simulink model "ADRC_DaoLiBai_test"  (R2018b)
settings: Solver=VariableStepAuto  StartTime=0.0  StopTime=10.0  RelTol=1e-3
settings Model: Creator=ILQMN  LastModifiedBy=ILQMN

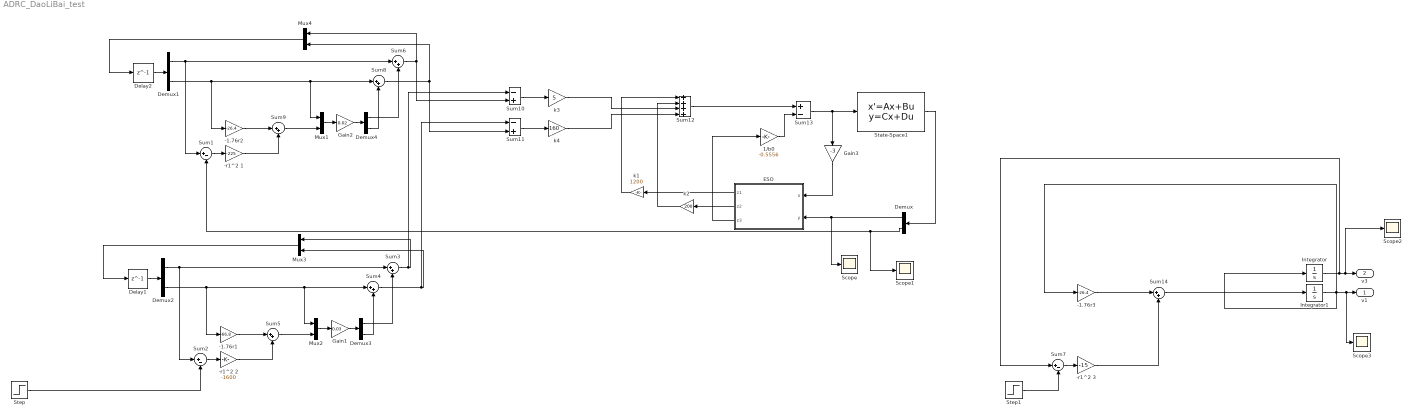
== system ADRC_DaoLiBai_test ==
  -1.76r1 : Gain  Gain=-66.8
  -1.76r2 : Gain  Gain=-26.4
  -1.76r3 : Gain  Gain=-26.4
  -r1^2 1 : Gain  Gain=-225
  -r1^2 2 : Gain  Gain=-1600
  -r1^2 3 : Gain  Gain=-15
  "1/b0 " : Gain  Gain=-0.5556
  Delay1 : Delay  DelayLength=1
  Delay2 : Delay  DelayLength=1
  Demux{,1..4} (5 alike) : Demux  Outputs=2
  ESO : Subsystem
  Gain1 : Gain  Gain=0.03
  Gain2 : Gain  Gain=0.02
  Gain3 : Gain  Gain=-3
  Integrator : Integrator
  Integrator1 : Integrator
  Mux{1..4} (4 alike) : Mux  Inputs=2
  Scope{,1..3} (4 alike) : Scope
  State-Space1 : StateSpace  A=[0 1 0 0;27.828 0 0 -0.2357;0 0 0 1;0.6393 0 0 -0.08832]  B=[0;2.6683;0;0.8832]  C=[1 0 0 0;0 0 1 0]  D=[0;0]  InitialCondition=[0;0;0;0]
  Step : Step  Time=2  After=0.2  SampleTime=0
  Step1 : Step  Time=0  SampleTime=0
  Sum1 : Sum  Inputs=|+-
  Sum10 : Sum  Inputs=-+
  Sum11 : Sum  Inputs=-+
  Sum12 : Sum  Inputs=++++
  Sum13 : Sum  Inputs=+-
  Sum{3..6,8..9,14} (7 alike) : Sum  Inputs=|++
  Sum2 : Sum  Inputs=|+-
  Sum7 : Sum  Inputs=|+-
  k1 : Gain  Gain=1200
  k2 : Gain  Gain=200
  k3 : Gain  Gain=5
  "k4 " : Gain  Gain=160
  v1 : Outport
  v3 : Outport  Port=2
  wires:
  Demux/1 -> Scope/1, ESO/2("y ")
  Sum12/1 -> Sum13/1
  Sum13/1 -> State-Space1/1, Gain3/1
  State-Space1/1 -> Demux/1
  "1/b0 "/1 -> Sum13/2
  k2/1 -> Sum12/2
  ESO/2(z2) -> k2/1
  "k4 "/1 -> Sum12/4
  k1/1 -> Sum12/1
  ESO/1(z1) -> k1/1
  k3/1 -> Sum12/3
  Sum10/1 -> k3/1
  Sum11/1 -> "k4 "/1
  ESO/3(z3) -> "1/b0 "/1
  Demux3/1 -> Sum3/2
  Delay1/1 -> Demux2/1
  Demux4/1 -> Sum6/2
  Demux3/2 -> Sum4/2
  Sum2/1 -> -r1^2 2/1
  Demux2/2 -> -1.76r1/1, Mux2/1, Sum4/1
  -1.76r1/1 -> Sum5/1
  Demux4/2 -> Sum8/2
  Demux2/1 -> Sum3/1, Sum2/1
  Delay2/1 -> Demux1/1
  Gain2/1 -> Demux4/1
  Step/1 -> Sum2/2
  Sum6/1 -> Sum10/2, Mux4/1
  Mux3/1 -> Delay1/1
  Sum3/1 -> Mux3/1, Sum10/1
  Demux1/1 -> Sum6/1, Sum1/1
  Demux1/2 -> -1.76r2/1, Mux1/1, Sum8/1
  Mux2/1 -> Gain1/1
  Sum1/1 -> -r1^2 1/1
  -1.76r2/1 -> Sum9/1
  Sum9/1 -> Mux1/2
  -r1^2 1/1 -> Sum9/2
  Sum5/1 -> Mux2/2
  Mux4/1 -> Delay2/1
  Sum4/1 -> Mux3/2, Sum11/1
  -r1^2 2/1 -> Sum5/2
  Gain1/1 -> Demux3/1
  Mux1/1 -> Gain2/1
  Demux/2 -> Scope1/1, Sum1/2
  Sum8/1 -> Sum11/2, Mux4/2
  Gain3/1 -> ESO/1("u ")
  -r1^2 3/1 -> Sum14/2
  Step1/1 -> Sum7/2
  Sum7/1 -> -r1^2 3/1
  -1.76r3/1 -> Sum14/1
  Integrator1/1 -> Integrator/1, Scope3/1, v1/1, -1.76r3/1
  Sum14/1 -> Integrator1/1
  Integrator/1 -> Sum7/1, Scope2/1, v3/1

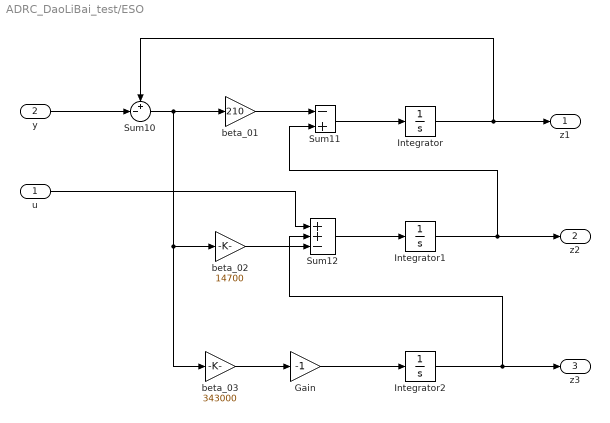
== system ADRC_DaoLiBai_test/ESO ==
  "u " : Inport
  "y " : Inport  Port=2
  Gain : Gain  Gain=-1
  Integrator : Integrator
  Integrator1 : Integrator
  Integrator2 : Integrator
  Sum10 : Sum  Inputs=+-|
  Sum11 : Sum  Inputs=-+
  Sum12 : Sum  Inputs=++-
  beta_01 : Gain  Gain=210
  beta_02 : Gain  Gain=14700
  beta_03 : Gain  Gain=343000
  z1 : Outport
  z2 : Outport  Port=2
  z3 : Outport  Port=3
  wires:
  beta_02/1 -> Sum12/3
  Gain/1 -> Integrator2/1
  Integrator1/1 -> Sum11/2, z2/1
  Integrator2/1 -> Sum12/2, z3/1
  Sum12/1 -> Integrator1/1
  "u "/1 -> Sum12/1
  beta_01/1 -> Sum11/1
  Sum10/1 -> beta_03/1, beta_02/1, beta_01/1
  Sum11/1 -> Integrator/1
  "y "/1 -> Sum10/2
  beta_03/1 -> Gain/1
  Integrator/1 -> z1/1, Sum10/1
